simulink model "CruiseControlModel"  (R2020b)
settings: Solver=VariableStepAuto  StartTime=0.0  StopTime=100  RelTol=1e-3
values from neighbouring files (symbols this model uses):
  b = 50.0    [CruiseControlData.sldd]
  m = 1000.0    [CruiseControlData.sldd]
settings Model: DataDictionary=CruiseControlData.sldd  Creator=Pavan  LastModifiedBy=Pavan
settings DataIOCC: SaveOutput=off  SaveTime=off

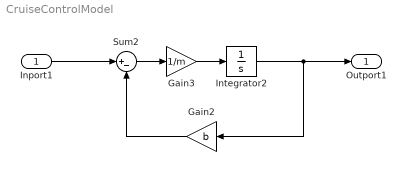
== system CruiseControlModel ==
  Inport1 : Inport
  Gain2 : Gain  Gain=b
  Gain3 : Gain  Gain=1/m
  Integrator2 : Integrator
  Sum2 : Sum  Inputs=|+-
  Outport1 : Outport
  wires:
  Gain3/1 -> Integrator2/1
  Sum2/1 -> Gain3/1
  Integrator2/1 -> Gain2/1, Outport1/1
  Inport1/1 -> Sum2/1
  Gain2/1 -> Sum2/2
